simulink model "drive_around"  (R2018a)
settings: Solver=FixedStepAuto  StartTime=0.0  StopTime=inf  FixedStep=sampleTime  RelTol=1e-3
PreLoadFcn:
  | driveParameters;
StopFcn:
  | saveMapToFile;
values from neighbouring files (symbols this model uses):
  angularGain = 1.5    [driveParameters.m]
  linearGain = 0.3    [driveParameters.m]
  mapUpdateTime = 5    [driveParameters.m]
  maxAngularRate = 1.5    [driveParameters.m]
  maxLinearRate = 0.5    [driveParameters.m]
undefined symbols (not defined in the file or in its folder): Angular, Linear
libraries: robotlib x3
settings Model: EnablePacing=on  Creator=scastro  LastModifiedBy=scastro
settings OptimizationCC: PassReuseOutputArgsAs=Individual arguments  MaxStackSize=64
settings DebuggingCC: ParameterTunabilityLossMsg=error
settings HardwareCC: ProdBitPerPointer=32  ProdBitPerSizeT=32  ProdBitPerPtrDiffT=32  ProdLargestAtomicFloat=None  ProdIntDivRoundTo=Undefined  ProdEndianess=Unspecified  ProdWordSize=32  ProdHWDeviceType=Generic->Unspecified (assume 32-bit Generic)
settings SFSimCC: MATLABDynamicMemAlloc=off
settings RTWCC: SystemTargetFile=ert.tlc  HardwareBoard=Robot Operating System (ROS)  TLCOptions="-aInlineSetEventsForThisBaseRateFcn=TLC_FALSE -aSuppressMultiTaskScheduler=TLC_FALSE  -aRateBasedStepFcn=0"  TemplateMakefile=ert_default_tmf  GenerateReport=on  Toolchain=Catkin  IncludeHyperlinkInReport=on  LaunchReport=on  TargetLang=C++  GenerateTraceInfo=on  GenerateTraceReport=on  GenerateTraceReportSl=on  GenerateTraceReportSf=on  GenerateTraceReportEml=on
settings CodeAppCC: ForceParamTrailComments=on  IgnoreCustomStorageClasses=off  OperatorAnnotations=on  SimulinkDataObjDesc=on  SFDataObjDesc=on  InsertBlockDesc=on

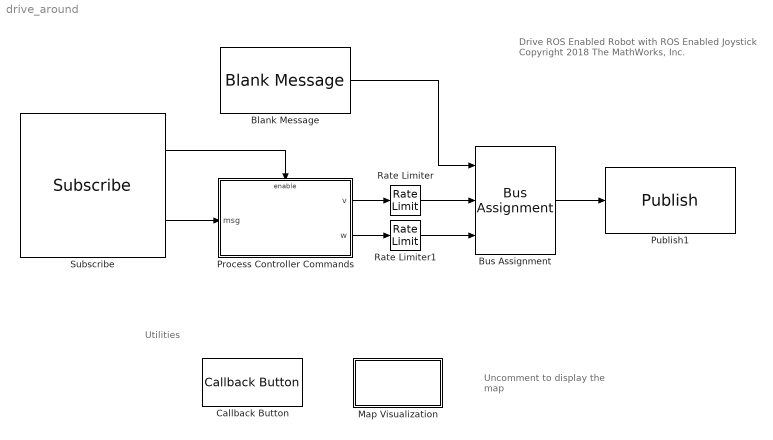
== system drive_around ==
  note: Drive ROS Enabled Robot with ROS Enabled Joystick
      |
      | Copyright 2018 The MathWorks, Inc.
  note: Utilities
  note: Uncomment to display the map
  Blank Message : robotlib/Blank Message  SourceLibraryInfo=This block requires Robotics System Toolbox  messageType=geometry_msgs/Twist  SampleTime=inf
      settings: SourceProductBaseCode=RO
  Bus Assignment : BusAssignment  DialogController=Simulink.DDGSource_BusAssignment  AssignedSignals=Linear.X,Angular.Z
  Callback Button : CallbackButton  WebBlockId=46  ButtonText=Save Map
      settings: ClickFcn=saveMapToFile;
  Map Visualization : Subsystem  mask(Map Visualization){Ts=mapUpdateTime}
      mask prompts: Ts "Sample Time"
      mask help:
      | Displays an occupancy grid received from the /map topic.
      |
      | The map updates based on the "Sample Time" parameter specified.
      mask Display: disp('Show Map')
  Process Controller Commands : Subsystem  TreatAsAtomicUnit=on
  Publish1 : robotlib/Publish  SourceLibraryInfo=This block requires Robotics System Toolbox  topicSource=Select from ROS network  topic=/mobile_base/commands/velocity  messageType=geometry_msgs/Twist  messageQueueLength=105
      settings: SourceProductBaseCode=RO
  Rate Limiter : RateLimiter  RisingSlewLimit=maxLinearRate  FallingSlewLimit=-maxLinearRate  SampleTimeMode=inherited
  Rate Limiter1 : RateLimiter  RisingSlewLimit=maxAngularRate  FallingSlewLimit=-maxAngularRate  SampleTimeMode=inherited
  Subscribe : robotlib/Subscribe  SourceLibraryInfo=This block requires Robotics System Toolbox  topicSource=Select from ROS network  topic=/joy  messageType=sensor_msgs/Joy  sampleTime=sampleTime  messageQueueLength=1
      settings: SourceProductBaseCode=RO
  wires:
  Subscribe/1 -> Process Controller Commands/Enable
  Subscribe/2 -> Process Controller Commands/1(msg)
  Bus Assignment/1 -> Publish1/1
  Process Controller Commands/2(w) -> Rate Limiter1/1
  Process Controller Commands/1(v) -> Rate Limiter/1
  Blank Message/1 -> Bus Assignment/1
  Rate Limiter/1 -> Bus Assignment/2
  Rate Limiter1/1 -> Bus Assignment/3

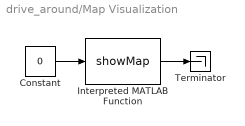
== system drive_around/Map Visualization ==
  Constant : Constant  Value=0  SampleTime=Ts
  Interpreted MATLAB Function : MATLABFcn  MATLABFcn=showMap
  Terminator : Terminator
  wires:
  Interpreted MATLAB Function/1 -> Terminator/1
  Constant/1 -> Interpreted MATLAB Function/1

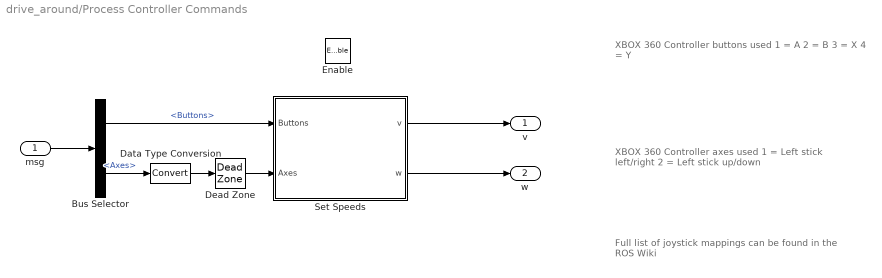
== system drive_around/Process Controller Commands ==
  note: Full list of joystick mappings can be found in the ROS Wiki
  note: XBOX 360 Controller buttons used
      | 1 = A
      | 2 = B
      | 3 = X
      | 4 = Y
  note: XBOX 360 Controller axes used
      | 1 = Left stick left/right
      | 2 = Left stick up/down
  msg : Inport
  Enable : EnablePort  StatesWhenEnabling=reset
  Bus Selector : BusSelector  OutputSignals=Buttons,Axes
  Data Type Conversion : DataTypeConversion
  Dead Zone : DeadZone  LowerValue=-0.1  UpperValue=0.1  SaturateOnIntegerOverflow=on
  Set Speeds : Stateflow chart  TreatAsAtomicUnit=on
  v : Outport
  w : Outport  Port=2
  wires:
  msg/1 -> Bus Selector/1
  Bus Selector/1 -> Set Speeds/1(Buttons)  "<Buttons>"
  Bus Selector/2 -> Data Type Conversion/1  "<Axes>"
  Data Type Conversion/1 -> Dead Zone/1
  Set Speeds/1(v) -> v/1
  Set Speeds/2(w) -> w/1
  Dead Zone/1 -> Set Speeds/2(Axes)

== stateflow chart drive_around/Process Controller Commands/Set Speeds ==
  (default) -> (junction 25) : % Unpack buttons into local variables
      | {
      | A = Buttons(1);
      | B = Buttons(2);
      | X = Buttons(3);
      | Y = Buttons(4);
      | }
  (junction 25) -> (junction 27) : % Proportional control based on joystick input
      | {
      | w = angularGain*Axes(1);
      | v = linearGain*Axes(2);
      | }
  (junction 27) -> (junction 28) [order 1] : [A || X] %If A or X is pressed, linear velocity only
  (junction 27) -> (junction 29) [order 2]
  (junction 28) -> (junction 30) : {w = 0;}
  (junction 30) -> (junction 29)
  (junction 29) -> (junction 47)
  (junction 47) -> (junction 44) [order 1] : [B || X] % If B or X is pressed, angular velocity only
  (junction 47) -> (junction 48) [order 2]
  (junction 44) -> (junction 34) : {v = 0;}
  (junction 34) -> (junction 48)
  (junction 48) -> (junction 84)
  (junction 84) -> (junction 82) [order 1] : [Y] % If Y is pressed, go half speed
  (junction 84) -> (junction 85) [order 2]
  (junction 82) -> (junction 87) : {
      | v = v/2;
      | w = w/2;
      | }
  (junction 87) -> (junction 85)
  data: v output; Buttons input; Axes input; w output; A local; X local; B local; angularGain parameter; linearGain parameter; Y local
